simulink model "QAM"  (R2020b)
settings: Solver=VariableStepAuto  StartTime=0.0  StopTime=200  RelTol=1e-3
libraries: simulink x14, dspsrcs4 x1, commchan3 x1, dspstat3 x1, dspsigops x1, commutil2 x1
(part 1 of 2)
settings Model: Creator=cxp10  LastModifiedBy=三三

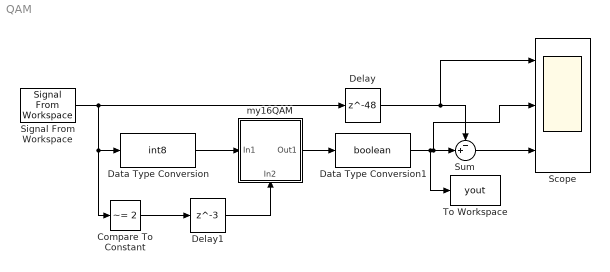
== system QAM ==
  Compare To Constant : simulink/Logic and Bit Operations/Compare To Constant  relop=~=  const=2  OutDataTypeStr=boolean
  Data Type Conversion : DataTypeConversion  OutDataTypeStr=int8
  Data Type Conversion1 : DataTypeConversion  OutDataTypeStr=boolean
  Delay : Delay  DelayLength=48  InitialCondition=0  SampleTime=0.01/4
  Delay1 : Delay  DelayLength=3  InitialCondition=0  SampleTime=0.01
  Scope : Scope  NumInputPorts=3
  Signal From Workspace : dspsrcs4/Signal From Workspace  X=simin  Ts=0.0025  nsamps=1  OutputAfterFinalValue=Setting to zero  ignoreOrWarnInputAndFrameLengths=off  OutputFrames=off
  Sum : Sum  Inputs=-+|  AccumDataTypeStr=double  OutDataTypeStr=double
  To Workspace : ToWorkspace  VariableName=yout  SampleTime=-1
      settings: Save2DSignal=2-D array (concatenate along first dimension)
  my16QAM : Subsystem
      settings: PortSchema="{\"entries\":[{\"content\":{\"sides\":[{\"content\":{\"connectorIds\":[\"In1\"]},\"type\":\"ConnectorPlacement.EquallySpacedRectSide\",\"uuid\":\"334856f7-0435-4d2a-9505-d8ddabddb349\"},{\"content\":{\"connectorIds\":[\"Out1\"],\"side\":\"RIGHT\"},\"type\":\"ConnectorPlacement.EquallySpacedRectSide\",\"uuid\":\"e3f7a207-8233-4ece-b29f-ed21cdef778a\"},{\"content\":{\"connectorIds\":[],\"side\":\"TOP\"},\"type\":\"ConnectorPlacement.EquallySpacedRectSide\",\"uuid\":\"48fa222e-92dd-480e-8acd-782dd06b0e97\"},{\"content\":{\"connectorIds\":[\"In2\"],\"side\":\"BOTTOM\"},\"type\":\"ConnectorPlacement.EquallySpacedRectSide\",\"uuid\":\"6010e3a1-3b49-41db-b06b-464f465d515b\"}]},\"type\":\"ConnectorPlacement.EquallySpacedConnector\",\"uuid\":\"a6a42f79-31a1-4a1c-b7ab-381f799bd7e3\"}],\"packageUris\":[\"http://schema.mathworks.com/mf0/Connector/19700101\"],\"version\":\"1.0\"}"
  wires:
  Data Type Conversion1/1 -> Sum/2, Scope/2, To Workspace/1
  Delay/1 -> Sum/1, Scope/1
  Data Type Conversion/1 -> my16QAM/1(In1)
  Sum/1 -> Scope/3
  Signal From Workspace/1 -> Delay/1, Compare To Constant/1, Data Type Conversion/1
  my16QAM/1(Out1) -> Data Type Conversion1/1
  Compare To Constant/1 -> Delay1/1
  Delay1/1 -> my16QAM/2(In2)

== system QAM/my16QAM ==
  In1 : Inport
  In2 : Inport  Port=2
  16QAM_core : Subsystem
      settings: PortSchema="{\"entries\":[{\"content\":{\"sides\":[{\"content\":{\"connectorIds\":[\"In1\"]},\"type\":\"ConnectorPlacement.EquallySpacedRectSide\",\"uuid\":\"334856f7-0435-4d2a-9505-d8ddabddb349\"},{\"content\":{\"connectorIds\":[\"Out1\"],\"side\":\"RIGHT\"},\"type\":\"ConnectorPlacement.EquallySpacedRectSide\",\"uuid\":\"e3f7a207-8233-4ece-b29f-ed21cdef778a\"},{\"content\":{\"connectorIds\":[],\"side\":\"TOP\"},\"type\":\"ConnectorPlacement.EquallySpacedRectSide\",\"uuid\":\"48fa222e-92dd-480e-8acd-782dd06b0e97\"},{\"content\":{\"connectorIds\":[\"In2\"],\"side\":\"BOTTOM\"},\"type\":\"ConnectorPlacement.EquallySpacedRectSide\",\"uuid\":\"02dbe2e7-12e3-4e06-b2a1-9218ba1a1d85\"}]},\"type\":\"ConnectorPlacement.EquallySpacedConnector\",\"uuid\":\"a6a42f79-31a1-4a1c-b7ab-381f799bd7e3\"}],\"packageUris\":[\"http://schema.mathworks.com/mf0/Connector/R2020b\"],\"version\":\"1.0\"}"
  串转并 : Subsystem
  并转串 : Subsystem
  Out1 : Outport
  wires:
  并转串/1(Out1) -> Out1/1
  In1/1 -> 串转并/1(In1)
  串转并/1(Out1) -> 16QAM_core/1(In1)
  16QAM_core/1(Out1) -> 并转串/1(In1)
  In2/1 -> 16QAM_core/2(In2)

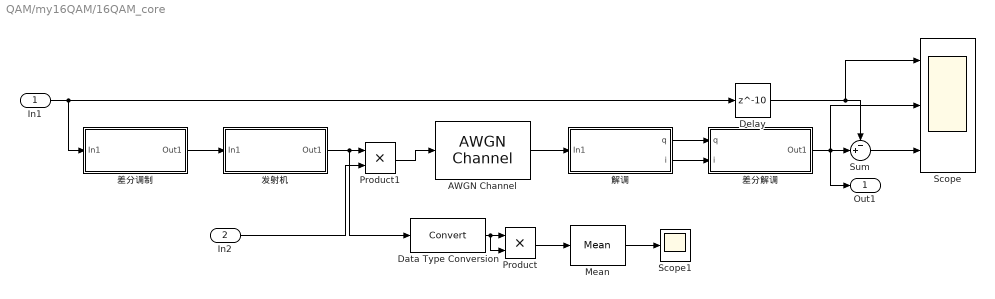
== system QAM/my16QAM/16QAM_core ==
  In1 : Inport
  In2 : Inport  Port=2
  AWGN Channel : commchan3/AWGN Channel  InputProcessing=Columns as channels (frame based)  seed=67  noiseMode="Signal to noise ratio  (SNR)"  EbNodB=10  EsNodB=10  SNRdB=12  bitsPerSym=1  Ps=0.0277  Tsym=1  variance=1
  Data Type Conversion : DataTypeConversion
  Delay : Delay  DelayLength=10  InitialCondition=0  SampleTime=0.01
  Mean : dspstat3/Mean  run=on  reset_popup=None  directionMode=Each column  dimension=1  roiEnable=off  roiType=Rectangles  roiPortion=Entire ROI  roiOutput=Individual statistics for each ROI  roiFlag=off  roundingMode=Floor  overflowMode=off  outputDataTypeStr=Inherit: Same as accumulator  outputMin=[]  outputMax=[]  outputLastDataTypeStr=Inherit: Same as accumulator
  Product : Product
  Product1 : Product
  Scope : Scope  NumInputPorts=3
  Scope1 : Scope
  Sum : Sum  Inputs=-+|  AccumDataTypeStr=double  OutDataTypeStr=double
  发射机 : Subsystem
  差分解调 : Subsystem
  差分调制 : Subsystem
  解调 : Subsystem
  Out1 : Outport
  wires:
  Delay/1 -> Sum/1, Scope/1
  Sum/1 -> Scope/3
  解调/1(q) -> 差分解调/1(q)
  解调/2(i) -> 差分解调/2(i)
  差分调制/1(Out1) -> 发射机/1(In1)
  AWGN Channel/1 -> 解调/1(In1)
  差分解调/1(Out1) -> Sum/2, Scope/2, Out1/1
  In1/1 -> Delay/1, 差分调制/1(In1)
  Product/1 -> Mean/1
  Mean/1 -> Scope1/1
  Data Type Conversion/1 -> Product/2, Product/1
  发射机/1(Out1) -> Data Type Conversion/1, Product1/1
  In2/1 -> Product1/2
  Product1/1 -> AWGN Channel/1

== system QAM/my16QAM/串转并 ==
  In1 : Inport
  Delay : Delay  InitialCondition=0  SampleTime=0.01/4
  Delay1 : Delay  DelayLength=3  InitialCondition=0  SampleTime=0.01/4
  Delay2 : Delay  DelayLength=4  InitialCondition=0  SampleTime=0.01/4
  Delay3 : Delay  DelayLength=1  InitialCondition=0  SampleTime=0.01
  Delay4 : Delay  DelayLength=1  InitialCondition=0  SampleTime=0.01/4
  Gain : Gain  Gain=2
  Gain1 : Gain  Gain=4
  Gain2 : Gain  Gain=8
  Sum : Sum  Inputs=++++
  Out1 : Outport
  wires:
  Delay4/1 -> Sum/1
  Delay3/1 -> Out1/1
  Delay/1 -> Gain/1
  Delay1/1 -> Gain1/1
  Gain2/1 -> Sum/4
  Sum/1 -> Delay3/1
  Gain1/1 -> Sum/3
  Delay2/1 -> Gain2/1
  Gain/1 -> Sum/2
  In1/1 -> Delay2/1, Delay1/1, Delay/1, Delay4/1

== system QAM/my16QAM/并转串 ==
  In1 : Inport
  Counter Limited : simulink/Sources/Counter Limited  uplimit=3  tsamp=0.01/4
  Data Type Conversion : DataTypeConversion  OutDataTypeStr=fixdt(0,4,0)
  Demux : Demux
      settings: DisplayOption=none
  Index Vector : MultiPortSwitch  DataPortOrder=Zero-based contiguous  Inputs=4  zeroidx=on
  Integer to Bit Converter : commutil2/Integer to Bit Converter  nbits=4  signedInputValues=Unsigned  bitOrder=MSB first  outDtype=Inherit via internal rule
  Out1 : Outport
  wires:
  Data Type Conversion/1 -> Integer to Bit Converter/1
  In1/1 -> Data Type Conversion/1
  Demux/3 -> Index Vector/4
  Integer to Bit Converter/1 -> Demux/1
  Demux/1 -> Index Vector/2
  Counter Limited/1 -> Index Vector/1
  Index Vector/1 -> Out1/1
  Demux/2 -> Index Vector/3
  Demux/4 -> Index Vector/5

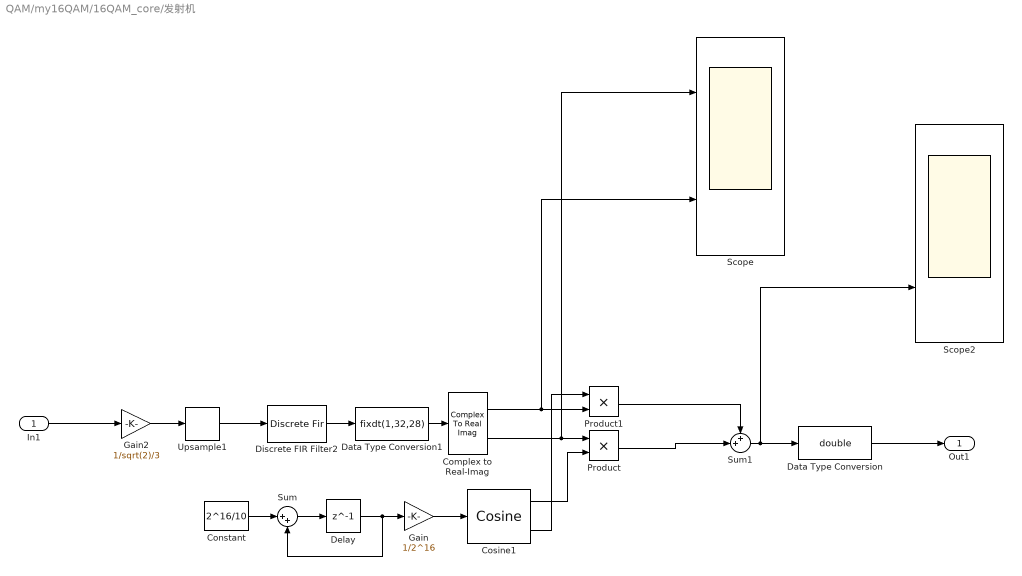
== system QAM/my16QAM/16QAM_core/发射机 ==
  In1 : Inport
  Complex to Real-Imag : ComplexToRealImag
  Constant : Constant  Value=2^16/10
  Cosine1 : simulink/Lookup Tables/Cosine  Formula=sin(2*pi*u) and cos(2*pi*u)  NumDataPoints=(2^16)+1  OutputWordLength=64  InternalRulePriority=Speed
      settings: SourceProductBaseCode=SL
  Data Type Conversion : DataTypeConversion  OutDataTypeStr=double
  Data Type Conversion1 : DataTypeConversion  OutDataTypeStr=fixdt(1,32,28)
  Delay : Delay  DelayLength=1  InitialCondition=0  SampleTime=0.001
  Discrete FIR Filter2 : DiscreteFir  Coefficients="[-0.0119566381847077\t-0.00554510890605436\t0.00241382573479933\t0.0111377436911783\t0.0196550101509641\t0.0268984171784200\t0.0318197882559029\t0.0335144832609033\t0.0313427539687735\t0.0250342434675171\t0.0147627477015526\t0.00118065713392810\t-0.0145939012931128\t-0.0310396234166703\t-0.0463415853998726\t-0.0585399944060724\t-0.0657057782491950\t-0.0661271775764019\t-0.0584895064408425\t-0.0420300071775653\t-0.0166513371647630\t0.0170194127981232\t0.0576344468660987\t0.103194189964349\t0.151177600592001\t0.198723997532092\t0.242851288478347\t0.280691625053822\t0.309723438717717\t0.327978774042235\t0.334206860938013\t0.327978774042235\t0.309723438717717\t0.280691625053822\t0.242851288478347\t0.198723997532092\t0.151177600592001\t0.103194189964349\t0.0576344468660987\t0.0170194127981232\t-0.0166513371647630\t-0.0420300071775653\t-0.0584895064408425\t-0.0661271775764019\t-0.0657057782491950\t-0.0585399944060724\t-0.0463415853998726\t-0.0310396234166703\t-0.0145939012931128\t0.00118065713392810\t0.0147627477015526\t0.0250342434675171\t0.0313427539687735\t0.0335144832609033\t0.0318197882559029\t0.0268984171784200\t0.0196550101509641\t0.0111377436911783\t0.00241382573479933\t-0.00554510890605436\t-0.0119566381847077]"
  Gain : Gain  Gain=1/2^16
  Gain2 : Gain  Gain=1/sqrt(2)/3  OutDataTypeStr=fixdt(1,32,28)
  Product : Product  OutDataTypeStr=fixdt(1,32,28)
  Product1 : Product  OutDataTypeStr=fixdt(1,32,28)
  Scope : Scope  NumInputPorts=2
  Scope2 : Scope  NumInputPorts=2
  Sum : Sum  Inputs=|++  OutMin=[0]  OutMax=[2^16-1]  OutDataTypeStr=fixdt(0,32,16)
  Sum1 : Sum  Inputs=++|  OutDataTypeStr=fixdt(1,32,28)
  Upsample1 : dspsigops/Upsample  N=10  phase=0  RateOptions=Allow multirate processing  ic=0  mode=Unused parameter value
  Out1 : Outport
  wires:
  Delay/1 -> Gain/1, Sum/2
  Cosine1/1 -> Product/2
  Sum/1 -> Delay/1
  Constant/1 -> Sum/1
  Gain/1 -> Cosine1/1
  Product1/1 -> Sum1/1
  Product/1 -> Sum1/2
  Complex to Real-Imag/1 -> Scope/2, Product1/2
  Complex to Real-Imag/2 -> Scope/1, Product/1
  Upsample1/1 -> Discrete FIR Filter2/1
  Sum1/1 -> Data Type Conversion/1, Scope2/2
  Gain2/1 -> Upsample1/1
  Discrete FIR Filter2/1 -> Data Type Conversion1/1
  Cosine1/2 -> Product1/1
  Data Type Conversion1/1 -> Complex to Real-Imag/1
  In1/1 -> Gain2/1
  Data Type Conversion/1 -> Out1/1

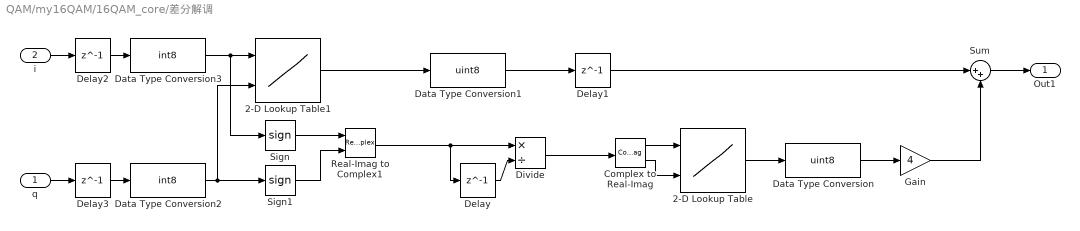
== system QAM/my16QAM/16QAM_core/差分解调 ==
  q : Inport
  i : Inport  Port=2
  2-D Lookup Table : Lookup_n-D  BreakpointsForDimension1=[-1 0 1]  BreakpointsForDimension2=[-1 0 1]  Table=[0 3 0;2 0 1;0 0 0]  ExtrapMethod=Clip  InternalRulePriority=Speed  RndMeth=Simplest  InputSameDT=on
      settings: InputPortMap=u0,u1
  2-D Lookup Table1 : Lookup_n-D  BreakpointsForDimension1=[-3 -1 1 3]  BreakpointsForDimension2=[-3 -1 1 3]  Table=[0 2 1 0; 1 3 3 2; 2 3 3 1; 0 1 2 0]  ExtrapMethod=Clip  InternalRulePriority=Speed  RndMeth=Simplest  InputSameDT=on
      settings: InputPortMap=u0,u1
  Complex to Real-Imag : ComplexToRealImag
  Data Type Conversion : DataTypeConversion  OutDataTypeStr=uint8
  Data Type Conversion1 : DataTypeConversion  OutDataTypeStr=uint8
  Data Type Conversion2 : DataTypeConversion  OutDataTypeStr=int8
  Data Type Conversion3 : DataTypeConversion  OutDataTypeStr=int8
  Delay{,1..3} (4 alike) : Delay  DelayLength=1  InitialCondition=1  SampleTime=0.01
  Divide : Product  Inputs=*/  OutDataTypeStr=int8
  Gain : Gain  Gain=4
  Real-Imag to Complex1 : RealImagToComplex
  Sign : Signum
  Sign1 : Signum
  Sum : Sum  Inputs=|++
  Out1 : Outport
  wires:
  Data Type Conversion1/1 -> Delay1/1
  2-D Lookup Table1/1 -> Data Type Conversion1/1
  Complex to Real-Imag/2 -> 2-D Lookup Table/2
  Gain/1 -> Sum/2
  Data Type Conversion/1 -> Gain/1
  Sum/1 -> Out1/1
  2-D Lookup Table/1 -> Data Type Conversion/1
  Complex to Real-Imag/1 -> 2-D Lookup Table/1
  Data Type Conversion3/1 -> Sign/1, 2-D Lookup Table1/1
  Delay/1 -> Divide/2
  Sign1/1 -> Real-Imag to Complex1/2
  Sign/1 -> Real-Imag to Complex1/1
  i/1 -> Delay2/1
  q/1 -> Delay3/1
  Data Type Conversion2/1 -> 2-D Lookup Table1/2, Sign1/1
  Real-Imag to Complex1/1 -> Divide/1, Delay/1
  Divide/1 -> Complex to Real-Imag/1
  Delay1/1 -> Sum/1
  Delay2/1 -> Data Type Conversion3/1
  Delay3/1 -> Data Type Conversion2/1

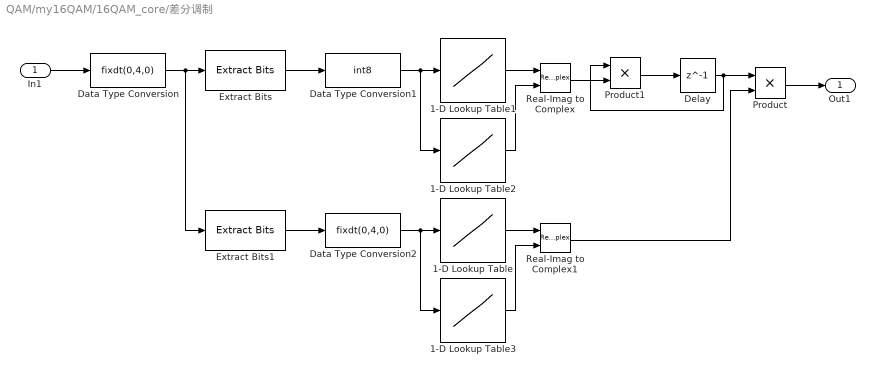
== system QAM/my16QAM/16QAM_core/差分调制 ==
  In1 : Inport
  1-D Lookup Table : Lookup_n-D  NumberOfTableDimensions=1  BreakpointsForDimension1=[0:3]  Table=[3 1 3 1]  ExtrapMethod=Clip  InternalRulePriority=Speed  RndMeth=Simplest  InputSameDT=on
  1-D Lookup Table1 : Lookup_n-D  NumberOfTableDimensions=1  BreakpointsForDimension1=[0:3]  Table=[1 0 0 -1]  ExtrapMethod=Clip  InternalRulePriority=Speed  RndMeth=Simplest  InputSameDT=on
  1-D Lookup Table2 : Lookup_n-D  NumberOfTableDimensions=1  BreakpointsForDimension1=[0:3]  Table=[0 1 -1 0]  ExtrapMethod=Clip  InternalRulePriority=Speed  RndMeth=Simplest  InputSameDT=on
  1-D Lookup Table3 : Lookup_n-D  NumberOfTableDimensions=1  BreakpointsForDimension1=[0:3]  Table=[3 3 1 1]  ExtrapMethod=Clip  InternalRulePriority=Speed  RndMeth=Simplest  InputSameDT=on
  Data Type Conversion : DataTypeConversion  OutDataTypeStr=fixdt(0,4,0)
  Data Type Conversion1 : DataTypeConversion  OutDataTypeStr=int8
  Data Type Conversion2 : DataTypeConversion  OutDataTypeStr=fixdt(0,4,0)
  Delay : Delay  DelayLength=1  InitialCondition=1  SampleTime=0.01
  Extract Bits : simulink/Logic and Bit Operations/Extract Bits  bitsToExtract=Upper half  numBits=2  bitIdxRange=[0 1]  outScalingMode=Treat bit field as an integer
  Extract Bits1 : simulink/Logic and Bit Operations/Extract Bits  bitsToExtract=Lower half  numBits=2  bitIdxRange=[0 1]  outScalingMode=Treat bit field as an integer
  Product : Product  OutDataTypeStr=fixdt(1,32,28)
  Product1 : Product  OutDataTypeStr=int8
  Real-Imag to Complex : RealImagToComplex
  Real-Imag to Complex1 : RealImagToComplex
  Out1 : Outport
  wires:
  Extract Bits1/1 -> Data Type Conversion2/1
  Product/1 -> Out1/1
  In1/1 -> Data Type Conversion/1
  1-D Lookup Table/1 -> Real-Imag to Complex1/1
  1-D Lookup Table1/1 -> Real-Imag to Complex/1
  Real-Imag to Complex1/1 -> Product/2
  1-D Lookup Table2/1 -> Real-Imag to Complex/2
  1-D Lookup Table3/1 -> Real-Imag to Complex1/2
  Product1/1 -> Delay/1
  Real-Imag to Complex/1 -> Product1/2
  Data Type Conversion2/1 -> 1-D Lookup Table/1, 1-D Lookup Table3/1
  Data Type Conversion1/1 -> 1-D Lookup Table1/1, 1-D Lookup Table2/1
  Data Type Conversion/1 -> Extract Bits1/1, Extract Bits/1
  Delay/1 -> Product/1, Product1/1
  Extract Bits/1 -> Data Type Conversion1/1

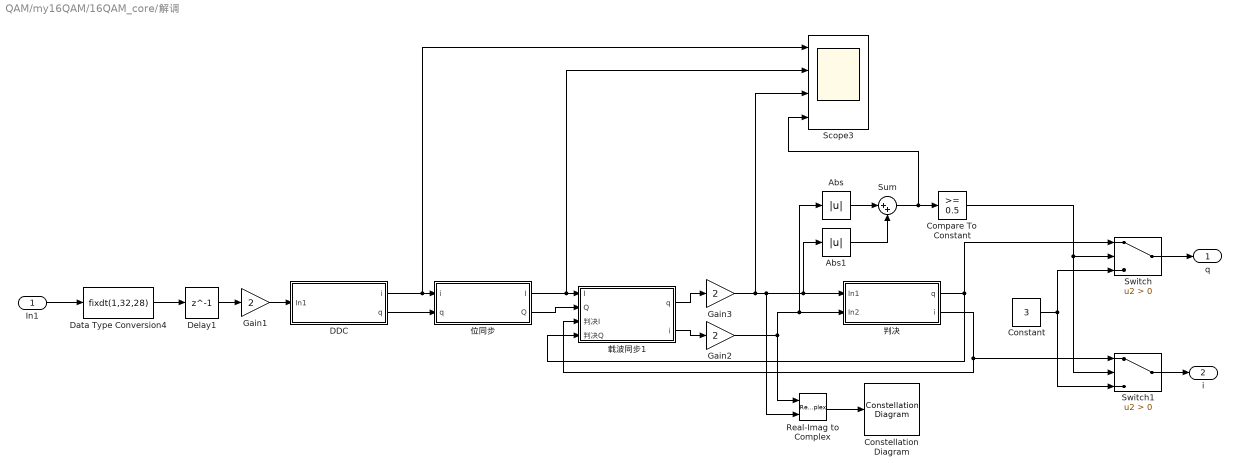
== system QAM/my16QAM/16QAM_core/解调 ==
  In1 : Inport
  Abs : Abs
  Abs1 : Abs
  Compare To Constant : simulink/Logic and Bit Operations/Compare To Constant  relop=>=  const=0.5  OutDataTypeStr=boolean
  Constant : Constant  Value=3  SampleTime=0.01
  Constellation Diagram : ConstellationDiagram
  DDC : Subsystem
  Data Type Conversion4 : DataTypeConversion  OutDataTypeStr=fixdt(1,32,28)
  Delay1 : Delay  DelayLength=1  InitialCondition=0  SampleTime=0.001
  Gain1 : Gain  Gain=2  OutDataTypeStr=fixdt(1,32,28)
  Gain2 : Gain  Gain=2  OutDataTypeStr=fixdt(1,32,28)
  Gain3 : Gain  Gain=2  OutDataTypeStr=fixdt(1,32,28)
  Real-Imag to Complex : RealImagToComplex
  Scope3 : Scope  NumInputPorts=4
  Sum : Sum  Inputs=|++  OutDataTypeStr=fixdt(1,32,28)
  Switch : Switch  Criteria=u2 > Threshold
  Switch1 : Switch  Criteria=u2 > Threshold
  位同步 : Subsystem
  判决 : Subsystem
  载波同步1 : Subsystem
  q : Outport
  i : Outport  Port=2
  wires:
  Data Type Conversion4/1 -> Delay1/1
  In1/1 -> Data Type Conversion4/1
  DDC/2(q) -> 位同步/2(q)
  Gain1/1 -> DDC/1(In1)
  DDC/1(i) -> Scope3/1, 位同步/1(i)
  位同步/2(Q) -> 载波同步1/2(Q)
  载波同步1/1(q) -> Gain3/1
  载波同步1/2(i) -> Gain2/1
  Real-Imag to Complex/1 -> Constellation Diagram/1
  位同步/1(I) -> Scope3/2, 载波同步1/1(I)
  判决/1(q) -> Switch/1, 载波同步1/4(判决Q)
  判决/2(i) -> Switch1/1, 载波同步1/3(判决I)
  Gain3/1 -> Real-Imag to Complex/2, Abs1/1, 判决/1(In1), Scope3/3
  Gain2/1 -> Abs/1, 判决/2(In2), Real-Imag to Complex/1
  Delay1/1 -> Gain1/1
  Abs/1 -> Sum/1
  Abs1/1 -> Sum/2
  Sum/1 -> Compare To Constant/1, Scope3/4
  Switch1/1 -> i/1
  Switch/1 -> q/1
  Compare To Constant/1 -> Switch1/2, Switch/2
  Constant/1 -> Switch1/3, Switch/3

== system QAM/my16QAM/16QAM_core/解调/DDC ==
  In1 : Inport
  Constant : Constant  Value=2^16/10
  Cosine : simulink/Lookup Tables/Cosine  Formula=cos(2*pi*u)  NumDataPoints=(2^16)+1  OutputWordLength=64  InternalRulePriority=Speed
      settings: SourceProductBaseCode=SL
  Cosine1 : simulink/Lookup Tables/Cosine  Formula=sin(2*pi*u)  NumDataPoints=(2^16)+1  OutputWordLength=64  InternalRulePriority=Speed
      settings: SourceProductBaseCode=SL
  Delay2 : Delay  DelayLength=1  InitialCondition=0  SampleTime=0.001
  Discrete FIR Filter3 : DiscreteFir  Coefficients="[-0.0119566381847077\t-0.00554510890605436\t0.00241382573479933\t0.0111377436911783\t0.0196550101509641\t0.0268984171784200\t0.0318197882559029\t0.0335144832609033\t0.0313427539687735\t0.0250342434675171\t0.0147627477015526\t0.00118065713392810\t-0.0145939012931128\t-0.0310396234166703\t-0.0463415853998726\t-0.0585399944060724\t-0.0657057782491950\t-0.0661271775764019\t-0.0584895064408425\t-0.0420300071775653\t-0.0166513371647630\t0.0170194127981232\t0.0576344468660987\t0.103194189964349\t0.151177600592001\t0.198723997532092\t0.242851288478347\t0.280691625053822\t0.309723438717717\t0.327978774042235\t0.334206860938013\t0.327978774042235\t0.309723438717717\t0.280691625053822\t0.242851288478347\t0.198723997532092\t0.151177600592001\t0.103194189964349\t0.0576344468660987\t0.0170194127981232\t-0.0166513371647630\t-0.0420300071775653\t-0.0584895064408425\t-0.0661271775764019\t-0.0657057782491950\t-0.0585399944060724\t-0.0463415853998726\t-0.0310396234166703\t-0.0145939012931128\t0.00118065713392810\t0.0147627477015526\t0.0250342434675171\t0.0313427539687735\t0.0335144832609033\t0.0318197882559029\t0.0268984171784200\t0.0196550101509641\t0.0111377436911783\t0.00241382573479933\t-0.00554510890605436\t-0.0119566381847077]"
  Discrete FIR Filter4 : DiscreteFir  Coefficients="[-0.0119566381847077\t-0.00554510890605436\t0.00241382573479933\t0.0111377436911783\t0.0196550101509641\t0.0268984171784200\t0.0318197882559029\t0.0335144832609033\t0.0313427539687735\t0.0250342434675171\t0.0147627477015526\t0.00118065713392810\t-0.0145939012931128\t-0.0310396234166703\t-0.0463415853998726\t-0.0585399944060724\t-0.0657057782491950\t-0.0661271775764019\t-0.0584895064408425\t-0.0420300071775653\t-0.0166513371647630\t0.0170194127981232\t0.0576344468660987\t0.103194189964349\t0.151177600592001\t0.198723997532092\t0.242851288478347\t0.280691625053822\t0.309723438717717\t0.327978774042235\t0.334206860938013\t0.327978774042235\t0.309723438717717\t0.280691625053822\t0.242851288478347\t0.198723997532092\t0.151177600592001\t0.103194189964349\t0.0576344468660987\t0.0170194127981232\t-0.0166513371647630\t-0.0420300071775653\t-0.0584895064408425\t-0.0661271775764019\t-0.0657057782491950\t-0.0585399944060724\t-0.0463415853998726\t-0.0310396234166703\t-0.0145939012931128\t0.00118065713392810\t0.0147627477015526\t0.0250342434675171\t0.0313427539687735\t0.0335144832609033\t0.0318197882559029\t0.0268984171784200\t0.0196550101509641\t0.0111377436911783\t0.00241382573479933\t-0.00554510890605436\t-0.0119566381847077]"
  Gain : Gain  Gain=1/2^16
  Gain1 : Gain  Gain=2  OutDataTypeStr=fixdt(1,32,28)
  Gain2 : Gain  Gain=2  OutDataTypeStr=fixdt(1,32,28)
  Product1 : Product  OutDataTypeStr=fixdt(1,32,28)
  Product2 : Product  OutDataTypeStr=fixdt(1,32,28)
  Sum1 : Sum  Inputs=|++  OutMin=[0]  OutMax=[2^16-1]  OutDataTypeStr=fixdt(0,32,16)
  i : Outport
  q : Outport  Port=2
  wires:
  Cosine1/1 -> Product2/2
  Constant/1 -> Sum1/1
  Sum1/1 -> Delay2/1
  Gain2/1 -> q/1
  Gain1/1 -> i/1
  Gain/1 -> Cosine/1, Cosine1/1
  Delay2/1 -> Sum1/2, Gain/1
  In1/1 -> Product1/2, Product2/1
  Cosine/1 -> Product1/1
  Discrete FIR Filter4/1 -> Gain1/1
  Product2/1 -> Discrete FIR Filter3/1
  Product1/1 -> Discrete FIR Filter4/1
  Discrete FIR Filter3/1 -> Gain2/1

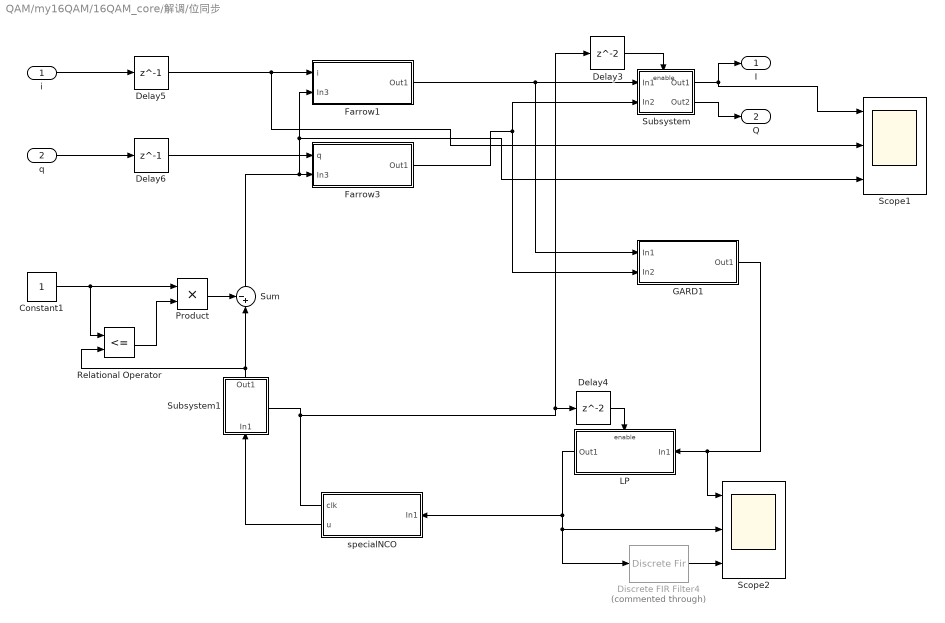
== system QAM/my16QAM/16QAM_core/解调/位同步 ==
  i : Inport
  q : Inport  Port=2
  Constant1 : Constant  OutDataTypeStr=fixdt(1,32,28)  SampleTime=0.01
  Delay3 : Delay  InitialCondition=0
  Delay4 : Delay  InitialCondition=0
  Delay5 : Delay  DelayLength=1  InitialCondition=0  SampleTime=0.001
  Delay6 : Delay  DelayLength=1  InitialCondition=0  SampleTime=0.001
  Discrete FIR Filter4 : DiscreteFir  Commented=through  Coefficients="[5.38827670327720e-05\t8.37859864059126e-06\t9.02577071280919e-06\t9.70599515144445e-06\t1.04165818557214e-05\t1.11621497031896e-05\t1.19399905979190e-05\t1.27547662205456e-05\t1.36038280216497e-05\t1.44919424768979e-05\t1.54165002359471e-05\t1.63821647738810e-05\t1.73863448370645e-05\t1.84338552877666e-05\t1.95220392829791e-05\t2.06555805408248e-05\t2.18322698177188e-05\t2.30558422383026e-05\t2.43269378472256e-05\t2.56438783973424e-05\t2.70139194785259e-05\t2.84325674352020e-05\t2.99013001451981e-05\t3.14273576150905e-05\t3.30048430841328e-05\t3.46380754777013e-05\t3.63271213027826e-05\t3.80773652938778e-05\t3.98849018394236e-05\t4.17539156292012e-05\t4.36830329961517e-05\t4.56781471467015e-05\t4.77366900846824e-05\t4.98628301063512e-05\t5.20540085491405e-05\t5.43152490247501e-05\t5.66456038712473e-05\t5.90491252349792e-05\t6.15249958158559e-05\t6.40756749798356e-05\t6.67003989259873e-05\t6.94040934711277e-05\t7.21842036194296e-05\t7.50467729337769e-05\t7.79894707634970e-05\t8.10163281991232e-05\t8.41252815914495e-05\t8.73216363738031e-05\t9.06029889739106e-05\t9.39743974468708e-05\t9.74342060955591e-05\t0.000100987692375075\t0.000104632192107747\t0.000108372281681474\t0.000112206342467372\t0.000116139266468525\t0.000120169404871481\t0.000124301052804280\t0.000128532823220613\t0.000132869575729040\t0.000137309181029465\t0.000141856789010187\t0.000146509847117926\t0.000151273286674838\t0.000156145642667454\t0.000161132018009352\t0.000166230083764592\t0.000171444733398769\t0.000176773605960749\t0.000182221612661642\t0.000187786593150612\t0.000193473629150883\t0.000199280488718983\t0.000205211685132340\t0.000211265398500019\t0.000217446507607164\t0.000223752761217449\t0.000230188784560116\t0.000236752520818625\t0.000243448735435774\t0.000250274983037235\t0.000257236019535067\t0.000264330100506618\t0.000271561990243754\t0.000278929355274878\t0.000286436890265331\t0.000294082033792734\t0.000301869596439394\t0.000309797345205324\t0.000317870189475281\t0.000326085384863677\t0.000334447075689439\t0.000342952903655544\t0.000351607352631286\t0.000360407616665803\t0.000369358318123430\t0.000378456801352178\t0.000387707364382725\t0.000397108082112494\t0.000406662934343845\t0.000416369204580440\t0.000426230755104286\t0.000436245388557304\t0.000446417742153065\t0.000456744884181980\t0.000467231199909950\t0.000477873972464166\t0.000488677251350832\t0.000499637440376430\t0.000510758673367827\t0.000522038396887917\t0.000533480280401991\t0.000545080769398471\t0.000556844103994101\t0.000568766185736806\t0.000580850432672023\t0.000593095234683480\t0.000605503378253917\t0.000618072781238363\t0.000630806222575761\t0.000643700780350444\t0.000656760471832712\t0.000669982400586430\t0.000683370025829815\t0.000696918573098365\t0.000710630926905871\t0.000724503829445785\t0.000738540917568113\t0.000752737001090627\t0.000767094386499337\t0.000781610766006477\t0.000796290631539730\t0.000811128092858480\t0.000826127681412666\t0.000841289250929616\t0.000856610300748781\t0.000872091884416860\t0.000887732449192652\t0.000903528018728126\t0.000919479373359454\t0.000935581446470775\t0.000951837298855666\t0.000968244039667702\t0.000984807285270455\t0.00100152517468790\t0.00101840099564402\t0.00103542695598586\t0.00105259888833481\t0.00106990529758374\t0.00108734964897944\t0.00110494267566542\t0.00112270934980982\t0.00114063129213466\t0.00115859990752069\t0.00117680222888921\t0.00119509959387189\t0.00121353986073303\t0.00123211546656185\t0.00125082134371779\t0.00126965953442028\t0.00128862434940582\t0.00130771774074139\t0.00132693385136779\t0.00134627449466985\t0.00136573389331197\t0.00138531384301694\t0.00140500830367386\t0.00142481894640172\t0.00144473975340373\t0.00146477179813887\t0.00148491072277744\t0.00150515201712332\t0.00152550251281669\t0.00154594432004887\t0.00156648817916740\t0.00158713046774516\t0.00160785883937208\t0.00162867840978680\t0.00164958598216596\t0.00167058052426799\t0.00169165284490608\t0.00171280423850651\t0.00173403000161468\t0.00175533174791612\t0.00177670178930184\t0.00179813963787842\t0.00181963802898036\t0.00184119812822650\t0.00186281437153346\t0.00188448678592134\t0.00190620967124911\t0.00192798028738096\t0.00194979411140008\t0.00197164956662192\t0.00199354018589733\t0.00201546789161710\t0.00203742463061031\t0.00205941027148300\t0.00208141816454080\t0.00210344802294037\t0.00212549178019049\t0.00214754993849286\t0.00216961587770786\t0.00219168966688694\t0.00221376332118668\t0.00223583683848542\t0.00225790312180091\t0.00227996159306796\t0.00230200480313444\t0.00232403181786743\t0.00234603631036743\t0.00236801777706385\t0.00238996920742478\t0.00241189033720393\t0.00243377280023632\t0.00245561659728671\t0.00247741441458659\t0.00249916562476833\t0.00252086247707472\t0.00254250471250362\t0.00256408444650458\t0.00258560151102332\t0.00260704842123784\t0.00262842494172428\t0.00264972299974808\t0.00267094199109233\t0.00269207461389840\t0.00271312023792777\t0.00273407126085464\t0.00275492724121749\t0.00277568079319803\t0.00279633128757952\t0.00281687073335238\t0.00283729896652871\t0.00285760864563827\t0.00287779930865078\t0.00289786332489527\t0.00291780003374124\t0.00293760134158108\t0.00295726700042838\t0.00297678944775037\t0.00299616850302645\t0.00301539634921388\t0.00303447287903666\t0.00305339092046008\t0.00307215012960474\t0.00309074294525690\t0.00310916914923290\t0.00312742099521662\t0.00314549848505173\t0.00316339462896414\t0.00318110881202524\t0.00319863347580294\t0.00321596813726239\t0.00323310586877002\t0.00325004654568439\t0.00326678292509291\t0.00328331562337832\t0.00329963761639421\t0.00331574889348412\t0.00333164194876551\t0.00334731729334170\t0.00336276794775731\t0.00337799391711069\t0.00339298833367161\t0.00340775154497468\t0.00342227577383967\t0.00343656199966569\t0.00345060427242355\t0.00346440245671541\t0.00347795086958273\t0.00349124911036735\t0.00350429126057300\t0.00351707814873492\t0.00352960351071997\t0.00354186762564742\t0.00355386316841616\t0.00356559141606362\t0.00357704675895919\t0.00358823039438686\t0.00359913555335254\t0.00360976414503881\t0.00362011126863201\t0.00363017742507951\t0.00363995506211021\t0.00364944695575173\t0.00365864686422917\t0.00366755392779621\t0.00367616707788512\t0.00368448516912521\t0.00369250555052204\t0.00370022882430508\t0.00370764908188711\t0.00371476694754616\t0.00372157637874722\t0.00372808046376311\t0.00373427584403981\t0.00374016638993305\t0.00374574619888750\t0.00375101445240137\t0.00375596347238067\t0.00376059842158154\t0.00376492136939815\t0.00376893584053243\t0.00377262402091522\t0.00377598540971720\t0.00377905127976721\t0.00378177794701704\t0.00378419317618726\t0.00378628656092737\t0.00378805733185340\t0.00378950843311406\t0.00379063573696286\t0.00379144285830933\t0.00379192563658652\t0.00379208785170762\t0.00379192563658652\t0.00379144285830933\t0.00379063573696286\t0.00378950843311406\t0.00378805733185340\t0.00378628656092737\t0.00378419317618726\t0.00378177794701704\t0.00377905127976721\t0.00377598540971720\t0.00377262402091522\t0.00376893584053243\t0.00376492136939815\t0.00376059842158154\t0.00375596347238067\t0.00375101445240137\t0.00374574619888750\t0.00374016638993305\t0.00373427584403981\t0.00372808046376311\t0.00372157637874722\t0.00371476694754616\t0.00370764908188711\t0.00370022882430508\t0.00369250555052204\t0.00368448516912521\t0.00367616707788512\t0.00366755392779621\t0.00365864686422917\t0.00364944695575173\t0.00363995506211021\t0.00363017742507951\t0.00362011126863201\t0.00360976414503881\t0.00359913555335254\t0.00358823039438686\t0.00357704675895919\t0.00356559141606362\t0.00355386316841616\t0.00354186762564742\t0.00352960351071997\t0.00351707814873492\t0.00350429126057300\t0.00349124911036735\t0.00347795086958273\t0.00346440245671541\t0.00345060427242355\t0.00343656199966569\t0.00342227577383967\t0.00340775154497468\t0.00339298833367161\t0.00337799391711069\t0.00336276794775731\t0.00334731729334170\t0.00333164194876551\t0.00331574889348412\t0.00329963761639421\t0.00328331562337832\t0.00326678292509291\t0.00325004654568439\t0.00323310586877002\t0.00321596813726239\t0.00319863347580294\t0.00318110881202524\t0.00316339462896414\t0.00314549848505173\t0.00312742099521662\t0.00310916914923290\t0.00309074294525690\t0.00307215012960474\t0.00305339092046008\t0.00303447287903666\t0.00301539634921388\t0.00299616850302645\t0.00297678944775037\t0.00295726700042838\t0.00293760134158108\t0.00291780003374124\t0.00289786332489527\t0.00287779930865078\t0.00285760864563827\t0.00283729896652871\t0.00281687073335238\t0.00279633128757952\t0.00277568079319803\t0.00275492724121749\t0.00273407126085464\t0.00271312023792777\t0.00269207461389840\t0.00267094199109233\t0.00264972299974808\t0.00262842494172428\t0.00260704842123784\t0.00258560151102332\t0.00256408444650458\t0.00254250471250362\t0.00252086247707472\t0.00249916562476833\t0.00247741441458659\t0.00245561659728671\t0.00243377280023632\t0.00241189033720393\t0.00238996920742478\t0.00236801777706385\t0.00234603631036743\t0.00232403181786743\t0.00230200480313444\t0.00227996159306796\t0.00225790312180091\t0.00223583683848542\t0.00221376332118668\t0.00219168966688694\t0.00216961587770786\t0.00214754993849286\t0.00212549178019049\t0.00210344802294037\t0.00208141816454080\t0.00205941027148300\t0.00203742463061031\t0.00201546789161710\t0.00199354018589733\t0.00197164956662192\t0.00194979411140008\t0.00192798028738096\t0.00190620967124911\t0.00188448678592134\t0.00186281437153346\t0.00184119812822650\t0.00181963802898036\t0.00179813963787842\t0.00177670178930184\t0.00175533174791612\t0.00173403000161468\t0.00171280423850651\t0.00169165284490608\t0.00167058052426799\t0.00164958598216596\t0.00162867840978680\t0.00160785883937208\t0.00158713046774516\t0.00156648817916740\t0.00154594432004887\t0.00152550251281669\t0.00150515201712332\t0.00148491072277744\t0.00146477179813887\t0.00144473975340373\t0.00142481894640172\t0.00140500830367386\t0.00138531384301694\t0.00136573389331197\t0.00134627449466985\t0.00132693385136779\t0.00130771774074139\t0.00128862434940582\t0.00126965953442028\t0.00125082134371779\t0.00123211546656185\t0.00121353986073303\t0.00119509959387189\t0.00117680222888921\t0.00115859990752069\t0.00114063129213466\t0.00112270934980982\t0.00110494267566542\t0.00108734964897944\t0.00106990529758374\t0.00105259888833481\t0.00103542695598586\t0.00101840099564402\t0.00100152517468790\t0.000984807285270455\t0.000968244039667702\t0.000951837298855666\t0.000935581446470775\t0.000919479373359454\t0.000903528018728126\t0.000887732449192652\t0.000872091884416860\t0.000856610300748781\t0.000841289250929616\t0.000826127681412666\t0.000811128092858480\t0.000796290631539730\t0.000781610766006477\t0.000767094386499337\t0.000752737001090627\t0.000738540917568113\t0.000724503829445785\t0.000710630926905871\t0.000696918573098365\t0.000683370025829815\t0.000669982400586430\t0.000656760471832712\t0.000643700780350444\t0.000630806222575761\t0.000618072781238363\t0.000605503378253917\t0.000593095234683480\t0.000580850432672023\t0.000568766185736806\t0.000556844103994101\t0.000545080769398471\t0.000533480280401991\t0.000522038396887917\t0.000510758673367827\t0.000499637440376430\t0.000488677251350832\t0.000477873972464166\t0.000467231199909950\t0.000456744884181980\t0.000446417742153065\t0.000436245388557304\t0.000426230755104286\t0.000416369204580440\t0.000406662934343845\t0.000397108082112494\t0.000387707364382725\t0.000378456801352178\t0.000369358318123430\t0.000360407616665803\t0.000351607352631286\t0.000342952903655544\t0.000334447075689439\t0.000326085384863677\t0.000317870189475281\t0.000309797345205324\t0.000301869596439394\t0.000294082033792734\t0.000286436890265331\t0.000278929355274878\t0.000271561990243754\t0.000264330100506618\t0.000257236019535067\t0.000250274983037235\t0.000243448735435774\t0.000236752520818625\t0.000230188784560116\t0.000223752761217449\t0.000217446507607164\t0.000211265398500019\t0.000205211685132340\t0.000199280488718983\t0.000193473629150883\t0.000187786593150612\t0.000182221612661642\t0.000176773605960749\t0.000171444733398769\t0.000166230083764592\t0.000161132018009352\t0.000156145642667454\t0.000151273286674838\t0.000146509847117926\t0.000141856789010187\t0.000137309181029465\t0.000132869575729040\t0.000128532823220613\t0.000124301052804280\t0.000120169404871481\t0.000116139266468525\t0.000112206342467372\t0.000108372281681474\t0.000104632192107747\t0.000100987692375075\t9.74342060955591e-05\t9.39743974468708e-05\t9.06029889739106e-05\t8.73216363738031e-05\t8.41252815914495e-05\t8.10163281991232e-05\t7.79894707634970e-05\t7.50467729337769e-05\t7.21842036194296e-05\t6.94040934711277e-05\t6.67003989259873e-05\t6.40756749798356e-05\t6.15249958158559e-05\t5.90491252349792e-05\t5.66456038712473e-05\t5.43152490247501e-05\t5.20540085491405e-05\t4.98628301063512e-05\t4.77366900846824e-05\t4.56781471467015e-05\t4.36830329961517e-05\t4.17539156292012e-05\t3.98849018394236e-05\t3.80773652938778e-05\t3.63271213027826e-05\t3.46380754777013e-05\t3.30048430841328e-05\t3.14273576150905e-05\t2.99013001451981e-05\t2.84325674352020e-05\t2.70139194785259e-05\t2.56438783973424e-05\t2.43269378472256e-05\t2.30558422383026e-05\t2.18322698177188e-05\t2.06555805408248e-05\t1.95220392829791e-05\t1.84338552877666e-05\t1.73863448370645e-05\t1.63821647738810e-05\t1.54165002359471e-05\t1.44919424768979e-05\t1.36038280216497e-05\t1.27547662205456e-05\t1.19399905979190e-05\t1.11621497031896e-05\t1.04165818557214e-05\t9.70599515144445e-06\t9.02577071280919e-06\t8.37859864059126e-06\t5.38827670327720e-05]"
  Farrow1 : Subsystem
  Farrow3 : Subsystem
  GARD1 : Subsystem
  LP : Subsystem
  Product : Product
  Relational Operator : RelationalOperator  Operator=<=  OutDataTypeStr=boolean  RndMeth=Simplest
  Scope1 : Scope  NumInputPorts=3
  Scope2 : Scope  NumInputPorts=3
  Subsystem : Subsystem
  Subsystem1 : Subsystem
  Sum : Sum  Inputs=-+|  OutDataTypeStr=fixdt(1,32,28)
  specialNCO : Subsystem
  I : Outport
  Q : Outport  Port=2
  wires:
  Farrow3/1(Out1) -> GARD1/2(In2), Subsystem/2(In2)
  Farrow1/1(Out1) -> GARD1/1(In1), Subsystem/1(In1)
  Subsystem/2(Out2) -> Q/1
  specialNCO/2(u) -> Subsystem1/1(In1)
  specialNCO/1(clk) -> Subsystem1/Enable, Delay3/1, Delay4/1
  LP/1(Out1) -> Discrete FIR Filter4/1, Scope2/2, specialNCO/1(In1)
  Delay3/1 -> Subsystem/Enable
  Delay4/1 -> LP/Enable
  GARD1/1(Out1) -> Scope2/1, LP/1(In1)
  Subsystem/1(Out1) -> Scope1/1, I/1
  i/1 -> Delay5/1
  q/1 -> Delay6/1
  Delay5/1 -> Scope1/2, Farrow1/1(i)
  Delay6/1 -> Farrow3/1(q)
  Discrete FIR Filter4/1 -> Scope2/3
  Subsystem1/1(Out1) -> Sum/2, Relational Operator/2
  Constant1/1 -> Relational Operator/1, Product/1
  Relational Operator/1 -> Product/2
  Product/1 -> Sum/1
  Sum/1 -> Farrow1/2(In3), Scope1/3, Farrow3/2(In3)

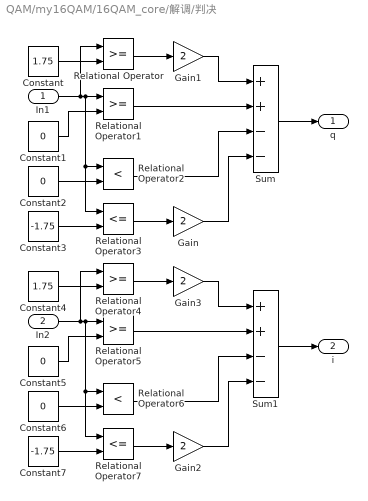
== system QAM/my16QAM/16QAM_core/解调/判决 ==
  In1 : Inport
  In2 : Inport  Port=2
  Constant : Constant  Value=1.75
  Constant{1..2,5..6} (4 alike) : Constant  Value=0
  Constant3 : Constant  Value=-1.75
  Constant4 : Constant  Value=1.75
  Constant7 : Constant  Value=-1.75
  Gain{,1..3} (4 alike) : Gain  Gain=2
  Relational Operator{,1,4..5} (4 alike) : RelationalOperator  OutDataTypeStr=boolean  RndMeth=Simplest
  Relational Operator2 : RelationalOperator  Operator=<  OutDataTypeStr=boolean  RndMeth=Simplest
  Relational Operator3 : RelationalOperator  Operator=<=  OutDataTypeStr=boolean  RndMeth=Simplest
  Relational Operator6 : RelationalOperator  Operator=<  OutDataTypeStr=boolean  RndMeth=Simplest
  Relational Operator7 : RelationalOperator  Operator=<=  OutDataTypeStr=boolean  RndMeth=Simplest
  Sum : Sum  Inputs=++--
  Sum1 : Sum  Inputs=++--
  q : Outport
  i : Outport  Port=2
  wires:
  Relational Operator2/1 -> Sum/3
  Sum/1 -> q/1
  Constant3/1 -> Relational Operator3/2
  Gain1/1 -> Sum/1
  Relational Operator3/1 -> Gain/1
  Gain/1 -> Sum/4
  Relational Operator1/1 -> Sum/2
  Relational Operator/1 -> Gain1/1
  Constant2/1 -> Relational Operator2/2
  Constant1/1 -> Relational Operator1/2
  Constant/1 -> Relational Operator/2
  In1/1 -> Relational Operator2/1, Relational Operator3/1, Relational Operator1/1, Relational Operator/1
  Gain2/1 -> Sum1/4
  Relational Operator7/1 -> Gain2/1
  Gain3/1 -> Sum1/1
  Constant7/1 -> Relational Operator7/2
  Sum1/1 -> i/1
  Relational Operator6/1 -> Sum1/3
  Constant5/1 -> Relational Operator5/2
  Constant6/1 -> Relational Operator6/2
  Relational Operator4/1 -> Gain3/1
  Relational Operator5/1 -> Sum1/2
  In2/1 -> Relational Operator6/1, Relational Operator7/1, Relational Operator5/1, Relational Operator4/1
  Constant4/1 -> Relational Operator4/2
